simulink model "NDT_Localization"  (R2022a)
settings: Solver=FixedStepAuto  StartTime=0.0  StopTime=10.0  RelTol=1e-3
model workspace (MAT data in the model file):
  SL_ROS_VariableLengthArrays_MaxSizes : object (value not decoded)
undefined symbols (not defined in the file or in its folder): null
libraries: ros2lib x9, robotlib x8, simulink x1
(part 2 of 12)

== system NDT_Localization/observation_callback/check_localizer/If Action Subsystem/register_measurement_impl/If Action Subsystem ==
  message_time : Inport
  ob_msg : Inport  Port=2
  ob_msg_data : Inport  Port=3
  initial_guess : Inport  Port=4
  m_map.frame_id() : Inport  Port=5
  m_map : Inport  Port=6
  localizer_ptr : Inport  Port=7
  Action Port : ActionPort  ActionPortLabel=if(u1 >= u2)
  If : If  IfExpression=u1 == 1  ShowElse=off
  If Action Subsystem : Subsystem  TreatAsAtomicUnit=on
  Merge : Merge
  validate_guess : Subsystem
  summary : Outport
  pose_out : Outport  Port=2
  Out1 : Outport  Port=3
  wires:
  message_time/1 -> If Action Subsystem/1(message_time), validate_guess/1(message_time)
  initial_guess/1 -> If Action Subsystem/2(initial_guess), validate_guess/2(initial_guess)
  validate_guess/1(Out1) -> Merge/1, If/1
  If/1 -> If Action Subsystem/Action
  ob_msg/1 -> If Action Subsystem/3(ob_msg)
  m_map/1 -> If Action Subsystem/5(m_map)
  m_map.frame_id()/1 -> If Action Subsystem/6(m_map.frame_id())
  ob_msg_data/1 -> If Action Subsystem/4(ob_msg_data)
  If Action Subsystem/1(summary) -> summary/1
  If Action Subsystem/2(pose_out) -> pose_out/1
  If Action Subsystem/3(Out2) -> Merge/2
  Merge/1 -> Out1/1
  localizer_ptr/1 -> If Action Subsystem/7(localizer_ptr)

== system NDT_Localization/observation_callback/check_localizer/If Action Subsystem/register_measurement_impl/If Action Subsystem1 ==
  Action Port : ActionPort  ActionPortLabel=else
  Constant : Constant  Value=0
  Out1 : Outport
  wires:
  Constant/1 -> Out1/1

== system NDT_Localization/observation_callback/check_localizer/If Action Subsystem/register_measurement_impl/validate_msg ==
  observation_time : Inport
  m_map : Inport  Port=2
  Add : Sum
  Bus Selector : BusSelector  OutputSignals=stamp.sec,stamp.nanosec
  Constant : Constant  Value=9
  If : If  NumInputs=2  IfExpression=u1 >= u2
  Math Function : Math  Operator=10^u
  Product : Product
  Out1 : Outport
  Out2 : Outport  Port=2
  wires:
  Add/1 -> If/2  "observation_time"
  Math Function/1 -> Product/2
  Constant/1 -> Math Function/1
  Product/1 -> Add/1
  Bus Selector/1 -> Product/1  "<sec>"
  observation_time/1 -> If/1
  Bus Selector/2 -> Add/2  "<nanosec>"
  m_map/1 -> Bus Selector/1
  If/2 -> Out2/1
  If/1 -> Out1/1

== system NDT_Localization/observation_callback/check_localizer/If Action Subsystem/validate_output/If Action Subsystem ==
  pose_out : Inport
  initial_guess : Inport  Port=2
  Action Port : ActionPort  ActionPortLabel=if(u1 ~= 0)
  Out1 : Outport
  wires:
  pose_out/1 -> Out1/1

== system NDT_Localization/observation_callback/check_localizer/If Action Subsystem/validate_output/If Action Subsystem1 ==
  pose_out : Inport
  initial_guess : Inport  Port=2
  Action Port : ActionPort  ActionPortLabel=if(u1 ~= 0)
  Out1 : Outport
  wires:
  pose_out/1 -> Out1/1

== system NDT_Localization/observation_callback/check_localizer/If Action Subsystem/validate_output/Switch Case Action Subsystem ==
  Action Port : ActionPort  ActionPortLabel=case [ 2 ]:
  ret_in : Constant  Value=false
  ret : Outport
  wires:
  ret_in/1 -> ret/1

== system NDT_Localization/observation_callback/check_localizer/If Action Subsystem/validate_output/Switch Case Action Subsystem1 ==
  summary : Inport
  pose_out : Inport  Port=2
  initial_guess : Inport  Port=3
  Action Port : ActionPort  ActionPortLabel=case [ 1 ]:
  Terminator : Terminator
  Terminator1 : Terminator
  Terminator2 : Terminator
  ret_in : Constant  Value=true
  ret : Outport
  wires:
  summary/1 -> Terminator/1
  pose_out/1 -> Terminator1/1
  initial_guess/1 -> Terminator2/1
  ret_in/1 -> ret/1

== system NDT_Localization/observation_callback/check_localizer/If Action Subsystem/validate_output/Switch Case Action Subsystem2 ==
  Action Port : ActionPort  ActionPortLabel=default:
  ret_in : Constant  Value=true
  ret : Outport
  wires:
  ret_in/1 -> ret/1

== system NDT_Localization/map_callback/check_localizer/set_map/set_map_impl/insert/insert_ ==
  msg : Inport
  If : If  NumInputs=2  IfExpression=u1 ~= 0 & u2 ~= 0
  If Action Subsystem : Subsystem  TreatAsAtomicUnit=on
  If Action Subsystem1 : Subsystem  TreatAsAtomicUnit=on
  Merge : Merge
  validate_pcl_map : Subsystem
  insert_res : Outport
  Out2 : Outport  Port=2
  wires:
  msg/1 -> validate_pcl_map/1(msg), If Action Subsystem/1(msg)
  validate_pcl_map/1(Out1) -> If/1
  If/1 -> If Action Subsystem/Action
  If Action Subsystem/1(insert_res) -> insert_res/1
  validate_pcl_map/2(offset) -> If Action Subsystem/2(offset)
  If/2 -> If Action Subsystem1/Action
  If Action Subsystem1/1(Out1) -> Merge/2
  If Action Subsystem/2(Out2) -> Merge/1
  Merge/1 -> Out2/1
  validate_pcl_map/3(ret) -> If/2

== system NDT_Localization/observation_callback/check_localizer/If Action Subsystem/If Action Subsystem/handle_registration_summary/If Action Subsystem ==
  summary : Inport
  Action Port : ActionPort  ActionPortLabel=if(u1 ~= 0)
  Publish : ros2lib/Publish  topicSource=Specify your own  topic=/increment_pub  messageType=sensor_msgs/PointCloud2  QOSHistory=Keep last  QOSDepth=1  QOSReliability=Reliable  QOSDurability=Volatile
      settings: SourceProductBaseCode=RR
  wires:
  summary/1 -> Publish/1

== system NDT_Localization/observation_callback/check_localizer/If Action Subsystem/guess/extrapolate/If Action Subsystem1 ==
  ret : Inport
  Action Port : ActionPort  ActionPortLabel=if(u1 ~= 0)
  Signal Conversion : SignalConversion  OverrideOpt=off
  Out2 : Outport
  wires:
  ret/1 -> Signal Conversion/1
  Signal Conversion/1 -> Out2/1

== system NDT_Localization/observation_callback/check_localizer/If Action Subsystem/guess/extrapolate/lookupTransform ==
  map_frame : Inport
  observation_frame : Inport  Port=2
  If : If  IfExpression=u1 ~= 0
  String Compare : StringCompare
  Switch : Switch  Criteria=u2 > Threshold  SaturateOnIntegerOverflow=off  InputSameDT=off
  TimePointZero : Constant  Value=0
  if_false : Subsystem  TreatAsAtomicUnit=on
  if_true : Subsystem  TreatAsAtomicUnit=on
  ret : Outport
  wires:
  Switch/1 -> ret/1
  map_frame/1 -> String Compare/1, if_false/1(target_frame), if_true/1(target_frame)
  if_true/1(identity) -> Switch/1
  TimePointZero/1 -> if_false/3(time), if_true/3(time)
  If/1 -> if_true/Action
  String Compare/1 -> Switch/2, If/1
  if_false/1(output_transform) -> Switch/3
  If/2 -> if_false/Action
  observation_frame/1 -> if_false/2(source_frame), if_true/2(source_frame), String Compare/2

== system NDT_Localization/observation_callback/check_localizer/If Action Subsystem/guess/lookupTransform/if_false ==
  target_frame : Inport
  source_frame : Inport  Port=2
  time : Inport  Port=3
  Action Port : ActionPort  ActionPortLabel=else
  Bus Creator : BusCreator  Inputs=3
  Bus Creator1 : BusCreator  Inputs=3
  Bus Creator2 : BusCreator  Inputs=2
  Bus Creator3 : BusCreator  Inputs=3
  Bus Creator4 : BusCreator  Inputs=4
  Bus Selector : BusSelector  OutputSignals=time,result_vec.x,result_vec.y,result_vec.z,result_quat.x,result_quat.y,result_quat.z,result_quat.w
  Constant : Constant
  Subsystem : Subsystem
  lookupFrameNumber : Subsystem
  lookupFrameNumber1 : Subsystem
  walkToTopParent : Subsystem  Commented=on
  output_transform : Outport
  wires:
  target_frame/1 -> lookupFrameNumber/1(target_frame), Bus Creator1/3  "frame_id"
  lookupFrameNumber/1(target_id) -> walkToTopParent/3(target_id)
  lookupFrameNumber1/1(source_id) -> walkToTopParent/4(source_id)
  time/1 -> walkToTopParent/2(time)
  Subsystem/1(accum) -> Bus Selector/1, walkToTopParent/1(accum)
  Constant/1 -> Bus Creator1/1  "sec"
  source_frame/1 -> Bus Creator/2, lookupFrameNumber1/1(source_frame)  "child_frame_id"
  Bus Selector/6 -> Bus Creator4/2  "<y>"
  Bus Creator3/1 -> Bus Creator2/1  "translation"
  Bus Selector/8 -> Bus Creator4/4  "<w>"
  Bus Creator4/1 -> Bus Creator2/2  "rotation"
  Bus Creator2/1 -> Bus Creator/3  "transform"
  Bus Creator1/1 -> Bus Creator/1  "header"
  Bus Selector/3 -> Bus Creator3/2  "<y>"
  Bus Selector/5 -> Bus Creator4/1  "<x>"
  Bus Selector/7 -> Bus Creator4/3  "<z>"
  Bus Creator/1 -> output_transform/1
  Bus Selector/1 -> Bus Creator1/2  "<time>"
  Bus Selector/2 -> Bus Creator3/1  "<x>"
  Bus Selector/4 -> Bus Creator3/3  "<z>"

== system NDT_Localization/observation_callback/check_localizer/If Action Subsystem/guess/lookupTransform/if_true ==
  target_frame : Inport
  source_frame : Inport  Port=2
  time : Inport  Port=3
  Action Port : ActionPort  ActionPortLabel=if(u1 ~= 0)
  Bus Creator : BusCreator  Inputs=3
  Bus Creator1 : BusCreator  Inputs=3
  Bus Creator2 : BusCreator  Inputs=2
  Bus Creator3 : BusCreator  Inputs=3
  Bus Creator4 : BusCreator  Inputs=4
  Constant : Constant  Value=false  OutDataTypeStr=boolean
  Current Time : robotlib/Current Time  Commented=on  OutputFormat=bus  SampleTime=-1  ModelName=NDT_Localization
      settings: SourceProductBaseCode=RR
  If : If  NumInputs=2  IfExpression=u1 == u2
  If Action Subsystem : Subsystem  TreatAsAtomicUnit=on
  If Action Subsystem1 : Subsystem  TreatAsAtomicUnit=on
  Merge : Merge
  Switch : Switch  Criteria=u2 > Threshold  SaturateOnIntegerOverflow=off  InputSameDT=off
  getFrame : Subsystem
  getLatestTimestamp : Subsystem
  lookupFrameNumber : Subsystem
  sec : Constant  Value=0  OutDataTypeStr=uint32
  w : Constant  OutDataTypeStr=single
  x : Constant  Value=0  OutDataTypeStr=single
  x1 : Constant  Value=0  OutDataTypeStr=single
  y : Constant  Value=0  OutDataTypeStr=single
  y1 : Constant  Value=0  OutDataTypeStr=single
  z : Constant  Value=0  OutDataTypeStr=single
  z1 : Constant  Value=0  OutDataTypeStr=single
  identity : Outport
  wires:
  Bus Creator1/1 -> Bus Creator/1  "header"
  sec/1 -> Bus Creator1/1  "sec"
  Bus Creator/1 -> identity/1
  source_frame/1 -> Bus Creator/2  "child_frame_id"
  Bus Creator2/1 -> Bus Creator/3  "transform"
  Bus Creator3/1 -> Bus Creator2/1  "translation"
  Bus Creator4/1 -> Bus Creator2/2  "rotation"
  Switch/1 -> Bus Creator1/2  "stamp"
  target_frame/1 -> Bus Creator1/3, lookupFrameNumber/1(target_frame)  "frame_id"
  x/1 -> Bus Creator3/1  "x"
  y/1 -> Bus Creator3/2  "y"
  z/1 -> Bus Creator3/3  "z"
  z1/1 -> Bus Creator4/3  "z"
  y1/1 -> Bus Creator4/2  "y"
  x1/1 -> Bus Creator4/1  "x"
  w/1 -> Bus Creator4/4  "w"
  time/1 -> Switch/3, If/1
  Current Time/1 -> If/2
  If/2 -> If Action Subsystem/Action
  If/1 -> If Action Subsystem1/Action
  If Action Subsystem1/1(out1) -> Merge/1
  If Action Subsystem/1(Out1) -> Merge/2
  Merge/1 -> Switch/2
  Constant/1 -> If Action Subsystem/1(In1)
  lookupFrameNumber/1(target_id) -> getFrame/1(target_id)
  getFrame/1(cache) -> If Action Subsystem1/1(cache), getLatestTimestamp/1(cache)
  getLatestTimestamp/1(LatestTimestamp) -> Switch/1

== system NDT_Localization/observation_callback/check_localizer/If Action Subsystem/register_measurement_impl/If Action Subsystem/If Action Subsystem ==
  message_time : Inport
  initial_guess : Inport  Port=2
  ob_msg : Inport  Port=3
  ob_msg_data : Inport  Port=4
  m_map : Inport  Port=5
  m_map.frame_id() : Inport  Port=6
  localizer_ptr : Inport  Port=7
  Action Port : ActionPort  ActionPortLabel=if(u1 == 1)
  Bus Creator : BusCreator  Inputs=3
  Bus Selector : BusSelector  OutputSignals=OptimizerT.optimizer_options,localizer_config.map_config.voxel_size.x,localizer_config.map_config.voxel_size.y,localizer_config.map_config.voxel_size.z,outlier_ratio
  Bus Selector3 : BusSelector  OutputSignals=transform
  Terminator : Terminator
  Terminator1 : Terminator
  insert : Subsystem
  solve : Subsystem
  transform_to_pose : Subsystem
  transform_to_pose1 : Subsystem
  summary : Outport
  pose_out : Outport  Port=2
  Out2 : Outport  Port=3
  wires:
  initial_guess/1 -> Bus Selector3/1
  Bus Selector3/1 -> transform_to_pose/1(transform_initial_transform)  "<transform>"
  ob_msg/1 -> Terminator/1, insert/2(ob_msg)
  message_time/1 -> insert/1(message_time)
  transform_to_pose/1(eig_pose_initial) -> solve/1(eig_pose_initial)
  insert/1(scan) -> Bus Creator/1  "scan"
  m_map/1 -> Bus Creator/2  "map"
  Bus Selector/5 -> solve/6(outlier_ratio)  "<outlier_ratio>"
  solve/1(summary) -> summary/1
  insert/2(Out2) -> Out2/1
  m_map.frame_id()/1 -> Terminator1/1
  Bus Creator/1 -> solve/2(problem)  "problem"
  ob_msg_data/1 -> insert/3(ob_msg_data)
  solve/2(eig_pose_out) -> transform_to_pose1/1(eig_pose_out)
  transform_to_pose1/1(pose_out.pose.pose) -> pose_out/1
  Bus Selector/2 -> solve/3(voxel_size_x)  "<x>"
  Bus Selector/3 -> solve/4(voxel_size_y)  "<y>"
  Bus Selector/4 -> solve/5(voxel_size_z)  "<z>"
  localizer_ptr/1 -> solve/7(localizer_ptr), Bus Selector/1
  Bus Selector/1 -> Bus Creator/3  "<optimizer_options>"

== system NDT_Localization/observation_callback/check_localizer/If Action Subsystem/register_measurement_impl/If Action Subsystem/validate_guess ==
  message_time : Inport
  initial_guess : Inport  Port=2
  Add : Sum  Inputs=++-  AccumDataTypeStr=uint64
  Bus Selector3 : BusSelector  OutputSignals=header.stamp.sec,header.stamp.nanosec
  Constant : Constant  Value=9
  If : If  NumInputs=2  IfExpression=u1 > u2
  If Action Subsystem : Subsystem  TreatAsAtomicUnit=on
  If Action Subsystem1 : Subsystem  TreatAsAtomicUnit=on
  Math Function : Math  Operator=10^u
  Merge : Merge
  Product : Product
  stamp_tol : Constant  Value=5000  OutDataTypeStr=uint64
  Out1 : Outport
  wires:
  initial_guess/1 -> Bus Selector3/1
  Bus Selector3/1 -> Product/1  "<sec>"
  Bus Selector3/2 -> Add/2  "<nanosec>"
  Product/1 -> Add/1
  Math Function/1 -> Product/2
  Constant/1 -> Math Function/1
  message_time/1 -> Add/3  "message_time"
  Add/1 -> If/1  "guess_scan_diff"
  stamp_tol/1 -> If/2
  If/1 -> If Action Subsystem/Action
  If/2 -> If Action Subsystem1/Action
  If Action Subsystem/1(Out1) -> Merge/1
  If Action Subsystem1/1(Out1) -> Merge/2
  Merge/1 -> Out1/1

== system NDT_Localization/map_callback/check_localizer/set_map/set_map_impl/insert/insert_/If Action Subsystem ==
  msg : Inport
  offset : Inport  Port=2
  Action Port : ActionPort  ActionPortLabel=if(u1 ~= 0)
  While Iterator Subsystem : Subsystem  TreatAsAtomicUnit=on
  insert_res : Outport
  Out2 : Outport  Port=2
  wires:
  msg/1 -> While Iterator Subsystem/1(msg)
  While Iterator Subsystem/1(insert_res) -> insert_res/1
  offset/1 -> While Iterator Subsystem/2(offset)
  While Iterator Subsystem/2(Out2) -> Out2/1

== system NDT_Localization/map_callback/check_localizer/set_map/set_map_impl/insert/insert_/If Action Subsystem1 ==
  Action Port : ActionPort  ActionPortLabel=else
  Constant : Constant  Value=0
  Out1 : Outport
  wires:
  Constant/1 -> Out1/1

== system NDT_Localization/map_callback/check_localizer/set_map/set_map_impl/insert/insert_/validate_pcl_map ==
  msg : Inport
  Add : Sum
  Add1 : Sum
  Add2 : Sum
  Bus Selector : BusSelector  OutputSignals=fields,point_step,height
  Cast : DataTypeConversion  OutDataTypeStr=int8  SaturateOnIntegerOverflow=off  RndMeth=Floor
  Compare To Constant : simulink/Logic and Bit Operations/Compare To Constant  relop=~=  const=1  OutDataTypeStr=boolean
  Constant : Constant  Value=-1
  Constant1 : Constant  Value=-2
  Gain : Gain  Gain=2
  If : If  IfExpression=u1 ~= 0
  If Action Subsystem : Subsystem  TreatAsAtomicUnit=on
  Logical Operator : Logic  Operator=OR  Inputs=3  AllPortsSameDT=off  OutDataTypeStr=boolean
  Merge : Merge
  Product : Product
  Relational Operator : RelationalOperator  Operator=~=  OutDataTypeStr=boolean  RndMeth=Simplest  InputSameDT=off
  Relational Operator1 : RelationalOperator  Operator=~=  OutDataTypeStr=boolean  RndMeth=Simplest  InputSameDT=off
  Width : Width  DataType=uint32
  check_fields : Subsystem  TreatAsAtomicUnit=on
  double_field_size : Constant  Value=8  OutDataTypeStr=uint32
  expected_num_fields : Constant  Value=10
  uint_field_size : Constant  Value=4  OutDataTypeStr=uint32
  Out1 : Outport
  offset : Outport  Port=2
  ret : Outport  Port=3
  wires:
  Bus Selector/1 -> check_fields/1(<fields>), Width/1  "<fields>"
  Logical Operator/1 -> Cast/1
  Product/1 -> Add/1
  double_field_size/1 -> Product/2, check_fields/2(double_field_size)
  Add1/1 -> Product/1
  msg/1 -> check_fields/4(msg), Bus Selector/1
  Bus Selector/3 -> Compare To Constant/1  "<height>"
  Compare To Constant/1 -> Logical Operator/3
  Bus Selector/2 -> Relational Operator1/1  "<point_step>"
  Width/1 -> Relational Operator/2
  Relational Operator1/1 -> Logical Operator/2
  expected_num_fields/1 -> Add2/1, Add1/1, Relational Operator/1
  uint_field_size/1 -> Gain/1
  Gain/1 -> Add/2
  Add/1 -> Relational Operator1/2
  Relational Operator/1 -> Logical Operator/1
  Merge/1 -> Out1/1
  Cast/1 -> If/1
  If/2 -> check_fields/Action
  If/1 -> If Action Subsystem/Action
  If Action Subsystem/1(Out1) -> Merge/1
  Constant/1 -> Add1/2
  Constant1/1 -> Add2/2
  Add2/1 -> check_fields/3(double_field_idx)  "double_field_idx"
  check_fields/1(Out1) -> Merge/2
  check_fields/2(offset) -> offset/1
  check_fields/3(ret) -> ret/1

== system NDT_Localization/observation_callback/check_localizer/If Action Subsystem/guess/extrapolate/lookupTransform/if_false ==
  target_frame : Inport
  source_frame : Inport  Port=2
  time : Inport  Port=3
  Action Port : ActionPort  ActionPortLabel=else
  Bus Creator : BusCreator  Inputs=3
  Bus Creator1 : BusCreator  Inputs=3
  Bus Creator2 : BusCreator  Inputs=2
  Bus Creator3 : BusCreator  Inputs=3
  Bus Creator4 : BusCreator  Inputs=4
  Bus Selector : BusSelector  OutputSignals=time,result_vec.x,result_vec.y,result_vec.z,result_quat.x,result_quat.y,result_quat.z,result_quat.w
  Constant : Constant
  Subsystem : Subsystem
  lookupFrameNumber : Subsystem
  lookupFrameNumber1 : Subsystem
  walkToTopParent : Subsystem  Commented=on
  output_transform : Outport
  wires:
  target_frame/1 -> lookupFrameNumber/1(target_frame), Bus Creator1/3  "frame_id"
  lookupFrameNumber/1(target_id) -> walkToTopParent/3(target_id)
  lookupFrameNumber1/1(source_id) -> walkToTopParent/4(source_id)
  time/1 -> walkToTopParent/2(time)
  Subsystem/1(accum) -> Bus Selector/1, walkToTopParent/1(accum)
  Constant/1 -> Bus Creator1/1  "sec"
  source_frame/1 -> Bus Creator/2, lookupFrameNumber1/1(source_frame)  "child_frame_id"
  Bus Selector/6 -> Bus Creator4/2  "<y>"
  Bus Creator3/1 -> Bus Creator2/1  "translation"
  Bus Selector/8 -> Bus Creator4/4  "<w>"
  Bus Creator4/1 -> Bus Creator2/2  "rotation"
  Bus Creator2/1 -> Bus Creator/3  "transform"
  Bus Creator1/1 -> Bus Creator/1  "header"
  Bus Selector/3 -> Bus Creator3/2  "<y>"
  Bus Selector/5 -> Bus Creator4/1  "<x>"
  Bus Selector/7 -> Bus Creator4/3  "<z>"
  Bus Creator/1 -> output_transform/1
  Bus Selector/1 -> Bus Creator1/2  "<time>"
  Bus Selector/2 -> Bus Creator3/1  "<x>"
  Bus Selector/4 -> Bus Creator3/3  "<z>"

== system NDT_Localization/observation_callback/check_localizer/If Action Subsystem/guess/extrapolate/lookupTransform/if_true ==
  target_frame : Inport
  source_frame : Inport  Port=2
  time : Inport  Port=3
  Action Port : ActionPort  ActionPortLabel=if(u1 ~= 0)
  Bus Creator : BusCreator  Inputs=3
  Bus Creator1 : BusCreator  Inputs=3
  Bus Creator2 : BusCreator  Inputs=2
  Bus Creator3 : BusCreator  Inputs=3
  Bus Creator4 : BusCreator  Inputs=4
  Constant : Constant  Value=false  OutDataTypeStr=boolean
  Current Time : robotlib/Current Time  Commented=on  OutputFormat=bus  SampleTime=-1  ModelName=NDT_Localization
      settings: SourceProductBaseCode=RR
  If : If  NumInputs=2  IfExpression=u1 == u2
  If Action Subsystem : Subsystem  TreatAsAtomicUnit=on
  If Action Subsystem1 : Subsystem  TreatAsAtomicUnit=on
  Merge : Merge
  Switch : Switch  Criteria=u2 > Threshold  SaturateOnIntegerOverflow=off  InputSameDT=off
  getFrame : Subsystem
  getLatestTimestamp : Subsystem
  lookupFrameNumber : Subsystem
  sec : Constant  Value=0  OutDataTypeStr=uint32
  w : Constant  OutDataTypeStr=single
  x : Constant  Value=0  OutDataTypeStr=single
  x1 : Constant  Value=0  OutDataTypeStr=single
  y : Constant  Value=0  OutDataTypeStr=single
  y1 : Constant  Value=0  OutDataTypeStr=single
  z : Constant  Value=0  OutDataTypeStr=single
  z1 : Constant  Value=0  OutDataTypeStr=single
  identity : Outport
  wires:
  Bus Creator1/1 -> Bus Creator/1  "header"
  sec/1 -> Bus Creator1/1  "sec"
  Bus Creator/1 -> identity/1
  source_frame/1 -> Bus Creator/2  "child_frame_id"
  Bus Creator2/1 -> Bus Creator/3  "transform"
  Bus Creator3/1 -> Bus Creator2/1  "translation"
  Bus Creator4/1 -> Bus Creator2/2  "rotation"
  Switch/1 -> Bus Creator1/2  "stamp"
  target_frame/1 -> Bus Creator1/3, lookupFrameNumber/1(target_frame)  "frame_id"
  x/1 -> Bus Creator3/1  "x"
  y/1 -> Bus Creator3/2  "y"
  z/1 -> Bus Creator3/3  "z"
  z1/1 -> Bus Creator4/3  "z"
  y1/1 -> Bus Creator4/2  "y"
  x1/1 -> Bus Creator4/1  "x"
  w/1 -> Bus Creator4/4  "w"
  time/1 -> Switch/3, If/1
  Current Time/1 -> If/2
  If/2 -> If Action Subsystem/Action
  If/1 -> If Action Subsystem1/Action
  If Action Subsystem1/1(out1) -> Merge/1
  If Action Subsystem/1(Out1) -> Merge/2
  Merge/1 -> Switch/2
  Constant/1 -> If Action Subsystem/1(In1)
  lookupFrameNumber/1(target_id) -> getFrame/1(target_id)
  getFrame/1(cache) -> If Action Subsystem1/1(cache), getLatestTimestamp/1(cache)
  getLatestTimestamp/1(LatestTimestamp) -> Switch/1

== system NDT_Localization/observation_callback/check_localizer/If Action Subsystem/guess/lookupTransform/if_false/Subsystem ==
  Bus Creator : BusCreator  Inputs=8
  Bus Creator1 : BusCreator  Inputs=5
  Bus Creator{2,4,6,9} (4 alike) : BusCreator  Inputs=4  OutDataTypeStr=Bus: SL_Bus_geometry_msgs_Quaternion
      settings: InheritFromInputs=off
  Bus Creator{3,5,7..8} (4 alike) : BusCreator  Inputs=3  OutDataTypeStr=Bus: SL_Bus_geometry_msgs_Vector3
      settings: InheritFromInputs=off
  Constant : Constant  OutDataTypeStr=uint32
  Constant1 : Constant  OutDataTypeStr=uint32
  Current Time : robotlib/Current Time  Commented=on  OutputFormat=bus  SampleTime=-1  ModelName=robotlib
      settings: SourceProductBaseCode=RR
  Current Time1 : robotlib/Current Time  Commented=on  OutputFormat=bus  SampleTime=-1  ModelName=robotlib
      settings: SourceProductBaseCode=RR
  w{,1..3} (4 alike) : Constant  OutDataTypeStr=single
  x{,1..7} (8 alike) : Constant  Value=0  OutDataTypeStr=single
  y{,1..7} (8 alike) : Constant  Value=0  OutDataTypeStr=single
  z{,1..7} (8 alike) : Constant  Value=0  OutDataTypeStr=single
  accum : Outport
  wires:
  Bus Creator3/1 -> Bus Creator/4  "source_to_top_vec"
  z4/1 -> Bus Creator6/3  "z"
  z7/1 -> Bus Creator9/3  "z"
  y7/1 -> Bus Creator9/2  "y"
  z1/1 -> Bus Creator4/3  "z"
  y6/1 -> Bus Creator8/2  "y"
  z3/1 -> Bus Creator5/3  "z"
  y1/1 -> Bus Creator4/2  "y"
  w3/1 -> Bus Creator9/4  "w"
  Constant1/1 -> Bus Creator1/5  "child_frame_id_"
  z6/1 -> Bus Creator8/3  "z"
  w/1 -> Bus Creator4/4  "w"
  y/1 -> Bus Creator3/2  "y"
  Bus Creator5/1 -> Bus Creator/6  "terget_to_top_vec"
  y3/1 -> Bus Creator5/2  "y"
  x6/1 -> Bus Creator8/1  "x"
  y4/1 -> Bus Creator6/2  "y"
  Bus Creator6/1 -> Bus Creator/7  "result_quat"
  Bus Creator1/1 -> Bus Creator/1  "st"
  Current Time/1 -> Bus Creator/2  "time"
  x7/1 -> Bus Creator9/1  "x"
  Bus Creator8/1 -> Bus Creator1/2  "translation_"
  Constant/1 -> Bus Creator1/4  "frame_id_"
  y2/1 -> Bus Creator2/2  "y"
  w2/1 -> Bus Creator6/4  "w"
  z2/1 -> Bus Creator2/3  "z"
  Bus Creator4/1 -> Bus Creator/3  "source_to_top_quat"
  x1/1 -> Bus Creator4/1  "x"
  x4/1 -> Bus Creator6/1  "x"
  z/1 -> Bus Creator3/3  "z"
  y5/1 -> Bus Creator7/2  "y"
  x2/1 -> Bus Creator2/1  "x"
  x5/1 -> Bus Creator7/1  "x"
  z5/1 -> Bus Creator7/3  "z"
  Bus Creator7/1 -> Bus Creator/8  "result_vec"
  w1/1 -> Bus Creator2/4  "w"
  x/1 -> Bus Creator3/1  "x"
  Bus Creator2/1 -> Bus Creator/5  "target_to_top_quat"
  Bus Creator9/1 -> Bus Creator1/1  "rotation_"
  Bus Creator/1 -> accum/1  "accum"
  x3/1 -> Bus Creator5/1  "x"
  Current Time1/1 -> Bus Creator1/3  "stamp_"

== system NDT_Localization/observation_callback/check_localizer/If Action Subsystem/guess/lookupTransform/if_false/lookupFrameNumber ==
  target_frame : Inport
  Cast : DataTypeConversion  OutDataTypeStr=uint32  SaturateOnIntegerOverflow=off  RndMeth=Floor
  target_id : Outport
  wires:
  target_frame/1 -> Cast/1
  Cast/1 -> target_id/1

== system NDT_Localization/observation_callback/check_localizer/If Action Subsystem/guess/lookupTransform/if_false/lookupFrameNumber1 ==
  source_frame : Inport
  Cast : DataTypeConversion  OutDataTypeStr=uint32  SaturateOnIntegerOverflow=off  RndMeth=Floor
  source_id : Outport
  wires:
  Cast/1 -> source_id/1
  source_frame/1 -> Cast/1

== system NDT_Localization/observation_callback/check_localizer/If Action Subsystem/guess/lookupTransform/if_false/walkToTopParent ==
  accum : Inport
  time : Inport  Port=2
  target_id : Inport  Port=3
  source_id : Inport  Port=4
  Out1 : Outport

== system NDT_Localization/observation_callback/check_localizer/If Action Subsystem/guess/lookupTransform/if_true/If Action Subsystem ==
  In1 : Inport
  Action Port : ActionPort  ActionPortLabel=else
  Out1 : Outport
  wires:
  In1/1 -> Out1/1

== system NDT_Localization/observation_callback/check_localizer/If Action Subsystem/guess/lookupTransform/if_true/If Action Subsystem1 ==
  cache : Inport
  Action Port : ActionPort  ActionPortLabel=if(u1 == u2)
  Constant : Constant  Commented=on  Value=null
  Constant1 : Constant  Value=true  OutDataTypeStr=boolean
  Constant2 : Constant  Value=false  OutDataTypeStr=boolean
  If : If  NumInputs=2  IfExpression=u1 ~= u2
  If Action Subsystem : Subsystem  TreatAsAtomicUnit=on
  If Action Subsystem1 : Subsystem  TreatAsAtomicUnit=on
  Merge : Merge
  out1 : Outport
  wires:
  Constant/1 -> If/2
  If/1 -> If Action Subsystem/Action
  If/2 -> If Action Subsystem1/Action
  Constant1/1 -> If Action Subsystem/1(In1)
  Constant2/1 -> If Action Subsystem1/1(In1)
  If Action Subsystem/1(Out1) -> Merge/1
  If Action Subsystem1/1(Out1) -> Merge/2
  Merge/1 -> out1/1
  cache/1 -> If/1

== system NDT_Localization/observation_callback/check_localizer/If Action Subsystem/guess/lookupTransform/if_true/getFrame ==
  target_id : Inport
  cache : Outport
  wires:
  target_id/1 -> cache/1

== system NDT_Localization/observation_callback/check_localizer/If Action Subsystem/guess/lookupTransform/if_true/getLatestTimestamp ==
  cache : Inport
  LatestTimestamp : Outport
  wires:
  cache/1 -> LatestTimestamp/1

== system NDT_Localization/observation_callback/check_localizer/If Action Subsystem/guess/lookupTransform/if_true/lookupFrameNumber ==
  target_frame : Inport
  Cast : DataTypeConversion  OutDataTypeStr=uint32  SaturateOnIntegerOverflow=off  RndMeth=Floor
  target_id : Outport
  wires:
  target_frame/1 -> Cast/1
  Cast/1 -> target_id/1

== system NDT_Localization/observation_callback/check_localizer/If Action Subsystem/register_measurement_impl/If Action Subsystem/If Action Subsystem/insert ==
  message_time : Inport
  ob_msg : Inport  Port=2
  ob_msg_data : Inport  Port=3
  Bus Selector : BusSelector  OutputSignals=width
  Constant : Constant  Value=-3
  If : If  NumInputs=2  IfExpression=u1 <= u2
  If Action Subsystem : Subsystem  TreatAsAtomicUnit=on
  If Action Subsystem1 : Subsystem  TreatAsAtomicUnit=on
  Math Function : Math  Operator=10^u
  Merge : Merge
  Product : Product
  Terminator : Terminator
  m_points.capacity : Constant  Value=55000
  scan : Outport
  Out2 : Outport  Port=2
  wires:
  ob_msg/1 -> Bus Selector/1
  message_time/1 -> Product/1
  Math Function/1 -> Product/2
  Constant/1 -> Math Function/1
  Product/1 -> Terminator/1  "m_stamp"
  Bus Selector/1 -> If/1  "<width>"
  If/1 -> If Action Subsystem/Action
  m_points.capacity/1 -> If/2, If Action Subsystem/2(In2)
  If/2 -> If Action Subsystem1/Action
  If Action Subsystem/2(Out2) -> Merge/1
  If Action Subsystem1/1(Out1) -> Merge/2
  Merge/1 -> Out2/1
  If Action Subsystem/1(points) -> scan/1
  ob_msg_data/1 -> If Action Subsystem/1(ob_msg_data)

== system NDT_Localization/observation_callback/check_localizer/If Action Subsystem/register_measurement_impl/If Action Subsystem/If Action Subsystem/solve ==
  eig_pose_initial : Inport
  problem : Inport  Port=2
  voxel_size_x : Inport  Port=3
  voxel_size_y : Inport  Port=4
  voxel_size_z : Inport  Port=5
  outlier_ratio : Inport  Port=6
  localizer_ptr : Inport  Port=7
  Add : Sum  Inputs=+
  Bus Selector : BusSelector  OutputSignals=scan,map,optimizer_options
  Bus Selector1 : BusSelector  OutputSignals=vx.centroid,vx.inv_covariance
  Bus Selector2 : BusSelector  OutputSignals=gradient_tolerance,max_iterations
  For Iterator Subsystem : Subsystem  TreatAsAtomicUnit=on
  If : If  NumInputs=2  IfExpression=u1 <= u2
  If Action Subsystem : Subsystem  TreatAsAtomicUnit=on
  If Action Subsystem1 : Subsystem  TreatAsAtomicUnit=on
  Math Function : Math  Operator=square
  Max : MinMax  Function=max
  Merge1 : Merge
  Product{,1..22} (23 alike) : Product  Multiplication=Matrix(*)
  Terminator : Terminator
  angle_params : Subsystem
  gradient_angle : Subsystem
  hessian_angle : Subsystem
  is_valid_probability : Subsystem  Commented=on
  point_gradient : MATLAB Function  TreatAsAtomicUnit=on
  point_hessian : MATLAB Function  TreatAsAtomicUnit=on
  set_hessian : MATLAB Function  TreatAsAtomicUnit=on
  set_jacobian : MATLAB Function  TreatAsAtomicUnit=on
  summary : Outport
  eig_pose_out : Outport  Port=2
  wires:
  problem/1 -> If Action Subsystem1/1(problem), Bus Selector/1
  Bus Selector/1 -> Product9/1, Product20/1, Product22/1, Product21/1, Product19/1, Product18/1, Product17/1, Product16/1, Product15/1, Product14/1, Product13/1, Product12/1, Product11/1, Product10/1, Product8/1, Product7/1, Product6/1, Product5/1, Product4/1, Product3/1, Product2/1, Product1/1, Product/1, For Iterator Subsystem/1(data)  "<scan>"
  voxel_size_y/1 -> For Iterator Subsystem/6(voxel_size_y), If Action Subsystem1/8(voxel_size_y)
  voxel_size_x/1 -> For Iterator Subsystem/5(voxel_size_x), If Action Subsystem1/7(voxel_size_x)
  voxel_size_z/1 -> If Action Subsystem1/9(voxel_size_z), For Iterator Subsystem/7(voxel_size_z)
  Bus Selector/2 -> Bus Selector1/1  "<map>"
  Bus Selector1/1 -> For Iterator Subsystem/2(myu)  "<centroid>"
  Bus Selector1/2 -> For Iterator Subsystem/3(sigma)  "<inv_covariance>"
  set_jacobian/1(jacobian) -> For Iterator Subsystem/8(set_jacobian)
  point_gradient/1(hessian) -> For Iterator Subsystem/9(set_gradient)
  set_hessian/1(hessian) -> For Iterator Subsystem/10(set_hessian)
  point_hessian/1(hessian) -> For Iterator Subsystem/11(point_hessian)
  angle_params/1(params) -> hessian_angle/1(params), gradient_angle/1(params)
  gradient_angle/1(ga_a_out) -> Product/2
  eig_pose_initial/1 -> If Action Subsystem1/5(eig_pose), angle_params/1(pose)
  Product/1 -> point_gradient/1(ga_a)
  Product1/1 -> point_gradient/2(ga_b)
  Product2/1 -> point_gradient/3(ga_c)
  Product3/1 -> point_gradient/4(ga_d)
  Product4/1 -> point_gradient/5(ga_e)
  gradient_angle/2(ga_b_out) -> Product1/2
  gradient_angle/3(ga_c_out) -> Product2/2
  gradient_angle/4(ga_d_out) -> Product3/2
  gradient_angle/5(ga_e_out) -> Product4/2
  Product5/1 -> point_gradient/6(ga_f)
  gradient_angle/6(ga_f_out) -> Product5/2
  Product6/1 -> point_gradient/7(ga_g)
  gradient_angle/7(ga_g_out) -> Product6/2
  Product7/1 -> point_gradient/8(ga_h)
  gradient_angle/8(ga_h_out) -> Product7/2
  Product8/1 -> point_hessian/1(ha_a2)
  hessian_angle/1(ha_a2_out) -> Product8/2
  Product9/1 -> point_hessian/2(ha_a3)
  hessian_angle/2(ha_a3_out) -> Product9/2
  Product10/1 -> point_hessian/3(ha_b2)
  hessian_angle/3(ha_b2_out) -> Product10/2
  Product11/1 -> point_hessian/4(ha_b3)
  hessian_angle/4(ha_b3_out) -> Product11/2
  Product12/1 -> point_hessian/5(ha_c2)
  hessian_angle/5(ha_c2_out) -> Product12/2
  Product13/1 -> point_hessian/6(ha_c3)
  hessian_angle/6(ha_c3_out) -> Product13/2
  Product14/1 -> point_hessian/7(ha_d1)
  hessian_angle/7(ha_d1_out) -> Product14/2
  Product15/1 -> point_hessian/8(ha_d2)
  hessian_angle/8(ha_d2_out) -> Product15/2
  Product16/1 -> point_hessian/9(ha_d3)
  hessian_angle/9(ha_d3_out) -> Product16/2
  Product17/1 -> point_hessian/10(ha_e1)
  hessian_angle/10(ha_e1_out) -> Product17/2
  Product18/1 -> point_hessian/11(ha_e2)
  hessian_angle/11(ha_e2_out) -> Product18/2
  Product19/1 -> point_hessian/12(ha_e3)
  hessian_angle/12(ha_e3_out) -> Product19/2
  Product20/1 -> point_hessian/13(ha_f1)
  hessian_angle/13(ha_f1_out) -> Product20/2
  Product21/1 -> point_hessian/14(ha_f2)
  hessian_angle/14(ha_f2_out) -> Product21/2
  Product22/1 -> point_hessian/15(ha_f3)
  hessian_angle/15(ha_f3_out) -> Product22/2
  For Iterator Subsystem/2(jacobian_out) -> If Action Subsystem1/2(jacobian), Math Function/1, Max/1
  If/1 -> If Action Subsystem/Action
  If/2 -> If Action Subsystem1/Action
  Bus Selector/3 -> Bus Selector2/1  "<optimizer_options>"
  Bus Selector2/1 -> If/2  "<gradient_tolerance>"
  Math Function/1 -> Add/1
  Add/1 -> If Action Subsystem/1(jacobian)
  Max/1 -> If/1
  If Action Subsystem/1(Out1) -> Merge1/1
  If Action Subsystem1/1(summary) -> Merge1/2
  Merge1/1 -> summary/1
  Bus Selector2/2 -> If Action Subsystem1/4(Max_iter)  "<max_iterations>"
  For Iterator Subsystem/3(hessian_out) -> If Action Subsystem1/3(hessian)
  For Iterator Subsystem/1(score_out) -> Terminator/1
  outlier_ratio/1 -> If Action Subsystem1/6(outlier_ratio), For Iterator Subsystem/4(outlier_ratio)
  If Action Subsystem1/2(eig_pose_result) -> eig_pose_out/1
  localizer_ptr/1 -> If Action Subsystem1/10(localizer_ptr)

== system NDT_Localization/observation_callback/check_localizer/If Action Subsystem/register_measurement_impl/If Action Subsystem/If Action Subsystem/transform_to_pose ==
  transform_initial_transform : Inport
  Add{,1..2,5,7} (5 alike) : Sum
  Add3 : Sum  Inputs=+-
  Add4 : Sum  Inputs=+-
  Add6 : Sum  Inputs=+-
  Asin : Trigonometry  Operator=asin
  Atan1 : Trigonometry  Operator=atan2
  Atan2 : Trigonometry  Operator=atan2
  Bus Selector : BusSelector  OutputSignals=translation,quaternion
  Bus Selector1 : BusSelector  OutputSignals=quaternion_w,quaternion_x,quaternion_y,quaternion_z
  Bus Selector2 : BusSelector  OutputSignals=translation_x,translation_y,translation_z
  Constant : Constant  Value=-2
  Constant1 : Constant  Value=2
  Constant2 : Constant
  Constant3 : Constant  Value=57.3
  Constant4 : Constant  Value=-1
  Constant5 : Constant  Value=pi/180
  Display : Display
  Divide : Product  Inputs=**
  Divide1 : Product  Inputs=**
  Divide2 : Product  Inputs=**
  Matrix Concatenate : Concatenate  NumInputs=6  Mode=Multidimensional array
  Product{,1,7..8} (4 alike) : Product  Inputs=3
  Product{2..6,9..12} (9 alike) : Product
  Square{,1..3} (4 alike) : Math  Operator=square  SignedPower=on
  eig_pose_initial : Outport  VectorParamsAs1DForOutWhenUnconnected=off
  wires:
  Bus Selector2/1 -> Matrix Concatenate/1  "<translation_x>"
  Bus Selector2/2 -> Matrix Concatenate/2  "<translation_y>"
  Bus Selector2/3 -> Matrix Concatenate/3  "<translation_z>"
  Add2/1 -> Add3/1
  Add7/1 -> Atan1/2
  Add1/1 -> Product5/2
  Bus Selector1/2 -> Product8/3, Square2/1, Product3/1  "<quaternion_x>"
  Product11/1 -> Divide/1
  Product12/1 -> Divide2/1
  Product1/1 -> Add/2
  Product3/1 -> Add1/1
  Atan2/1 -> Product6/2
  Atan1/1 -> Product11/2
  Divide/1 -> Matrix Concatenate/4
  Product10/1 -> Add6/2
  Product4/1 -> Add1/2
  Bus Selector1/3 -> Product7/2, Square1/1, Product3/2, Product1/3  "<quaternion_y>"
  Constant4/1 -> Product12/2
  Product9/1 -> Add6/1
  Product8/1 -> Add5/2
  Product6/1 -> Product12/1
  Add/1 -> Asin/1
  Product5/1 -> Atan2/1
  Bus Selector1/1 -> Product8/2, Square3/1, Product4/1, Product1/2, Product/2  "<quaternion_w>"
  Bus Selector1/4 -> Product7/3, Square/1, Product4/2, Product/3  "<quaternion_z>"
  Constant1/1 -> Product8/1, Product7/1, Product10/1, Product5/1, Product1/1
  Add4/1 -> Atan2/2
  Constant/1 -> Product9/1, Product/1
  Constant3/1 -> Product2/1, Product6/1, Product11/1
  Product7/1 -> Add5/1
  Constant5/1 -> Divide/2, Divide2/2, Divide1/2
  Divide1/1 -> Matrix Concatenate/5
  Product2/1 -> Divide1/1
  Add3/1 -> Add4/1
  Divide2/1 -> Matrix Concatenate/6
  Add6/1 -> Add7/2
  Product/1 -> Add/1
  Square/1 -> Add4/2
  Asin/1 -> Product2/2
  Add5/1 -> Atan1/1
  Square2/1 -> Product9/2, Add2/2
  Constant2/1 -> Add7/1
  Square3/1 -> Add2/1
  Square1/1 -> Product10/2, Add3/2
  Matrix Concatenate/1 -> Display/1, eig_pose_initial/1
  transform_initial_transform/1 -> Bus Selector/1
  Bus Selector/2 -> Bus Selector1/1  "<quaternion>"
  Bus Selector/1 -> Bus Selector2/1  "<translation>"

== system NDT_Localization/observation_callback/check_localizer/If Action Subsystem/register_measurement_impl/If Action Subsystem/If Action Subsystem/transform_to_pose1 ==
  eig_pose_out : Inport
  Add{,1..2,5,7} (5 alike) : Sum
  Add3 : Sum  Inputs=+-
  Add4 : Sum  Inputs=+-
  Add6 : Sum  Inputs=+-
  Asin : Trigonometry  Operator=asin
  Atan1 : Trigonometry  Operator=atan2
  Atan2 : Trigonometry  Operator=atan2
  Bus Selector : BusSelector  OutputSignals=translation,quaternion
  Bus Selector1 : BusSelector  OutputSignals=quaternion_w,quaternion_x,quaternion_y,quaternion_z
  Bus Selector2 : BusSelector  OutputSignals=translation_x,translation_y,translation_z
  Constant : Constant  Value=-2
  Constant1 : Constant  Value=2
  Constant2 : Constant
  Constant3 : Constant  Value=57.3
  Constant4 : Constant  Value=-1
  Constant5 : Constant  Value=pi/180
  Display : Display
  Divide : Product  Inputs=**
  Divide1 : Product  Inputs=**
  Divide2 : Product  Inputs=**
  Matrix Concatenate : Concatenate  NumInputs=6  Mode=Multidimensional array
  Product{,1,7..8} (4 alike) : Product  Inputs=3
  Product{2..6,9..12} (9 alike) : Product
  Square{,1..3} (4 alike) : Math  Operator=square  SignedPower=on
  pose_out.pose.pose : Outport  VectorParamsAs1DForOutWhenUnconnected=off
  wires:
  Bus Selector2/1 -> Matrix Concatenate/1  "<translation_x>"
  Bus Selector2/2 -> Matrix Concatenate/2  "<translation_y>"
  Bus Selector2/3 -> Matrix Concatenate/3  "<translation_z>"
  Add2/1 -> Add3/1
  Add7/1 -> Atan1/2
  Add1/1 -> Product5/2
  Bus Selector1/2 -> Product8/3, Square2/1, Product3/1  "<quaternion_x>"
  Product11/1 -> Divide/1
  Product12/1 -> Divide2/1
  Product1/1 -> Add/2
  Product3/1 -> Add1/1
  Atan2/1 -> Product6/2
  Atan1/1 -> Product11/2
  Divide/1 -> Matrix Concatenate/4
  Product10/1 -> Add6/2
  Product4/1 -> Add1/2
  Bus Selector1/3 -> Product7/2, Square1/1, Product3/2, Product1/3  "<quaternion_y>"
  Constant4/1 -> Product12/2
  Product9/1 -> Add6/1
  Product8/1 -> Add5/2
  Product6/1 -> Product12/1
  Add/1 -> Asin/1
  Product5/1 -> Atan2/1
  Bus Selector1/1 -> Product8/2, Square3/1, Product4/1, Product1/2, Product/2  "<quaternion_w>"
  Bus Selector1/4 -> Product7/3, Square/1, Product4/2, Product/3  "<quaternion_z>"
  Constant1/1 -> Product8/1, Product7/1, Product10/1, Product5/1, Product1/1
  Add4/1 -> Atan2/2
  Constant/1 -> Product9/1, Product/1
  Constant3/1 -> Product2/1, Product6/1, Product11/1
  Product7/1 -> Add5/1
  Constant5/1 -> Divide/2, Divide2/2, Divide1/2
  Divide1/1 -> Matrix Concatenate/5
  Product2/1 -> Divide1/1
  Add3/1 -> Add4/1
  Divide2/1 -> Matrix Concatenate/6
  Add6/1 -> Add7/2
  Product/1 -> Add/1
  Square/1 -> Add4/2
  Asin/1 -> Product2/2
  Add5/1 -> Atan1/1
  Square2/1 -> Product9/2, Add2/2
  Constant2/1 -> Add7/1
  Square3/1 -> Add2/1
  Square1/1 -> Product10/2, Add3/2
  Matrix Concatenate/1 -> Display/1, pose_out.pose.pose/1
  eig_pose_out/1 -> Bus Selector/1
  Bus Selector/2 -> Bus Selector1/1  "<quaternion>"
  Bus Selector/1 -> Bus Selector2/1  "<translation>"

== system NDT_Localization/observation_callback/check_localizer/If Action Subsystem/register_measurement_impl/If Action Subsystem/validate_guess/If Action Subsystem ==
  Action Port : ActionPort  ActionPortLabel=if(u1 > u2)
  Constant : Constant  Value=0
  Out1 : Outport
  wires:
  Constant/1 -> Out1/1

== system NDT_Localization/observation_callback/check_localizer/If Action Subsystem/register_measurement_impl/If Action Subsystem/validate_guess/If Action Subsystem1 ==
  Action Port : ActionPort  ActionPortLabel=else
  Constant : Constant
  Out1 : Outport
  wires:
  Constant/1 -> Out1/1

== system NDT_Localization/map_callback/check_localizer/set_map/set_map_impl/insert/insert_/If Action Subsystem/While Iterator Subsystem ==
  msg : Inport
  offset : Inport  Port=2
  Add : Sum
  Bus Creator : BusCreator  Inputs=2
  Bus Selector : BusSelector  OutputSignals=row_step,point_step,header.stamp
  Constant : Constant
  Data Type Conversion : DataTypeConversion  OutDataTypeStr=uint8  SaturateOnIntegerOverflow=off  RndMeth=Floor
  Data Type Conversion{1..3,5..6,9} (6 alike) : DataTypeConversion  OutDataTypeStr=double  SaturateOnIntegerOverflow=off  RndMeth=Floor
  Delay : Delay  DelayLength=1
  If : If  IfExpression=u1 ~= 0
  If Action Subsystem : Subsystem  TreatAsAtomicUnit=on
  If Action Subsystem1 : Subsystem  TreatAsAtomicUnit=on
  MATLAB Function : MATLAB Function  TreatAsAtomicUnit=on
  MATLAB Function1 : MATLAB Function  TreatAsAtomicUnit=on
  MATLAB Function2 : MATLAB Function  TreatAsAtomicUnit=on
  Merge : Merge
  Read Point Cloud : ros2lib/Read Point Cloud  MaximumPointCloudSize=[480, 640]  PreserveStructure=off  ShowRGBOutput=off  ShowIntensityOutput=off  ShowErrorCodeOutput=off  VariableSizeOutputs=off
      settings: SourceProductBaseCode=RR
  Relational Operator : RelationalOperator  Operator=~=  OutDataTypeStr=boolean  RndMeth=Simplest  InputSameDT=off
  Relational Operator1 : RelationalOperator  Operator=~=  OutDataTypeStr=boolean  RndMeth=Simplest  InputSameDT=off
  Relational Operator2 : RelationalOperator  Operator===  OutDataTypeStr=boolean  RndMeth=Simplest  InputSameDT=off
  While Iterator : WhileIterator  MaxIters=55000  ShowIterationPort=on  OutputDataType=uint32
  index : Subsystem
  insert_res : Outport
  Out2 : Outport  Port=2
  wires:
  Relational Operator/1 -> While Iterator/2
  msg/1 -> MATLAB Function/1(msg), Bus Selector/1
  Bus Selector/1 -> Relational Operator/1, Relational Operator1/2  "<row_step>"
  Constant/1 -> Relational Operator/2, Add/2
  Relational Operator1/1 -> While Iterator/1
  While Iterator/1 -> Delay/1, MATLAB Function/2(id), Relational Operator2/2
  Add/1 -> Relational Operator1/1
  Delay/1 -> Add/1
  MATLAB Function/1(point) -> MATLAB Function1/1(point), Read Point Cloud/1
  Read Point Cloud/1 -> Bus Creator/1, index/1(pt)  "centroid"
  index/1(idx) -> If Action Subsystem/1(voxel_idx), Relational Operator2/1  "voxel_idx"
  Relational Operator2/1 -> Data Type Conversion/1
  Data Type Conversion/1 -> If/1
  If/1 -> If Action Subsystem/Action
  If Action Subsystem/1(insert_res) -> insert_res/1
  MATLAB Function2/1(inv_covariance) -> Bus Creator/2  "inv_covariance"
  Bus Creator/1 -> If Action Subsystem/2(vx)  "vx"
  offset/1 -> MATLAB Function1/3(offset)
  Bus Selector/2 -> MATLAB Function1/2(point_step)  "<point_step>"
  MATLAB Function1/1(xx) -> Data Type Conversion1/1
  Data Type Conversion1/1 -> MATLAB Function2/1(xx)
  MATLAB Function1/2(xy) -> Data Type Conversion2/1
  MATLAB Function1/3(xz) -> Data Type Conversion3/1
  MATLAB Function1/4(yy) -> Data Type Conversion5/1
  MATLAB Function1/5(yz) -> Data Type Conversion6/1
  MATLAB Function1/6(zz) -> Data Type Conversion9/1
  Data Type Conversion2/1 -> MATLAB Function2/2(xy)
  Data Type Conversion3/1 -> MATLAB Function2/3(xz)
  Data Type Conversion5/1 -> MATLAB Function2/4(yy)
  Data Type Conversion6/1 -> MATLAB Function2/5(yz)
  Data Type Conversion9/1 -> MATLAB Function2/6(zz)
  If/2 -> If Action Subsystem1/Action
  If Action Subsystem/2(Out2) -> Merge/1
  If Action Subsystem1/1(Out1) -> Merge/2
  Merge/1 -> Out2/1
  Bus Selector/3 -> If Action Subsystem/3(<stamp>)  "<stamp>"

== system NDT_Localization/map_callback/check_localizer/set_map/set_map_impl/insert/insert_/validate_pcl_map/If Action Subsystem ==
  Action Port : ActionPort  ActionPortLabel=if(u1 ~= 0)
  Constant : Constant  Value=0
  Out1 : Outport
  wires:
  Constant/1 -> Out1/1

== system NDT_Localization/map_callback/check_localizer/set_map/set_map_impl/insert/insert_/validate_pcl_map/check_fields ==
  <fields> : Inport
  double_field_size : Inport  Port=2
  double_field_idx : Inport  Port=3
  msg : Inport  Port=4
  Action Port : ActionPort  ActionPortLabel=else
  Cast : DataTypeConversion  OutDataTypeStr=int8  SaturateOnIntegerOverflow=off  RndMeth=Floor
  For Iterator Subsystem : Subsystem  TreatAsAtomicUnit=on
  If : If  IfExpression=u1 ~= 0
  If Action Subsystem : Subsystem  TreatAsAtomicUnit=on
  Logical Operator : Logic  Operator=OR  AllPortsSameDT=off  OutDataTypeStr=boolean
  Merge : Merge
  Subsystem : Subsystem
  Width : Width
  check_fields_name : Subsystem  TreatAsAtomicUnit=on
  Out1 : Outport
  offset : Outport  Port=2
  ret : Outport  Port=3
  wires:
  Logical Operator/1 -> Cast/1
  Cast/1 -> If/1
  If/2 -> check_fields_name/Action
  <fields>/1 -> Width/1, For Iterator Subsystem/2(<fields>), Subsystem/1(<fields>), check_fields_name/1(<fields>)
  If/1 -> If Action Subsystem/Action
  If Action Subsystem/1(Out1) -> Merge/1
  check_fields_name/1(Out1) -> Merge/2
  Merge/1 -> Out1/1
  Width/1 -> For Iterator Subsystem/1(In1)
  double_field_size/1 -> Subsystem/2(double_field_size), For Iterator Subsystem/3(double_field_size)
  double_field_idx/1 -> For Iterator Subsystem/4(double_field_idx)
  For Iterator Subsystem/1(Out1) -> Logical Operator/1
  Subsystem/1(Out1) -> Logical Operator/2
  msg/1 -> check_fields_name/2(msg)
  check_fields_name/2(offset) -> offset/1
  check_fields_name/3(ret) -> ret/1

== system NDT_Localization/observation_callback/check_localizer/If Action Subsystem/guess/extrapolate/lookupTransform/if_false/Subsystem ==
  Bus Creator : BusCreator  Inputs=8
  Bus Creator1 : BusCreator  Inputs=5
  Bus Creator{2,4,6,9} (4 alike) : BusCreator  Inputs=4  OutDataTypeStr=Bus: SL_Bus_geometry_msgs_Quaternion
      settings: InheritFromInputs=off
  Bus Creator{3,5,7..8} (4 alike) : BusCreator  Inputs=3  OutDataTypeStr=Bus: SL_Bus_geometry_msgs_Vector3
      settings: InheritFromInputs=off
  Constant : Constant  OutDataTypeStr=uint32
  Constant1 : Constant  OutDataTypeStr=uint32
  Current Time : robotlib/Current Time  Commented=on  OutputFormat=bus  SampleTime=-1  ModelName=robotlib
      settings: SourceProductBaseCode=RR
  Current Time1 : robotlib/Current Time  Commented=on  OutputFormat=bus  SampleTime=-1  ModelName=robotlib
      settings: SourceProductBaseCode=RR
  w{,1..3} (4 alike) : Constant  OutDataTypeStr=single
  x{,1..7} (8 alike) : Constant  Value=0  OutDataTypeStr=single
  y{,1..7} (8 alike) : Constant  Value=0  OutDataTypeStr=single
  z{,1..7} (8 alike) : Constant  Value=0  OutDataTypeStr=single
  accum : Outport
  wires:
  Bus Creator3/1 -> Bus Creator/4  "source_to_top_vec"
  z4/1 -> Bus Creator6/3  "z"
  z7/1 -> Bus Creator9/3  "z"
  y7/1 -> Bus Creator9/2  "y"
  z1/1 -> Bus Creator4/3  "z"
  y6/1 -> Bus Creator8/2  "y"
  z3/1 -> Bus Creator5/3  "z"
  y1/1 -> Bus Creator4/2  "y"
  w3/1 -> Bus Creator9/4  "w"
  Constant1/1 -> Bus Creator1/5  "child_frame_id_"
  z6/1 -> Bus Creator8/3  "z"
  w/1 -> Bus Creator4/4  "w"
  y/1 -> Bus Creator3/2  "y"
  Bus Creator5/1 -> Bus Creator/6  "terget_to_top_vec"
  y3/1 -> Bus Creator5/2  "y"
  x6/1 -> Bus Creator8/1  "x"
  y4/1 -> Bus Creator6/2  "y"
  Bus Creator6/1 -> Bus Creator/7  "result_quat"
  Bus Creator1/1 -> Bus Creator/1  "st"
  Current Time/1 -> Bus Creator/2  "time"
  x7/1 -> Bus Creator9/1  "x"
  Bus Creator8/1 -> Bus Creator1/2  "translation_"
  Constant/1 -> Bus Creator1/4  "frame_id_"
  y2/1 -> Bus Creator2/2  "y"
  w2/1 -> Bus Creator6/4  "w"
  z2/1 -> Bus Creator2/3  "z"
  Bus Creator4/1 -> Bus Creator/3  "source_to_top_quat"
  x1/1 -> Bus Creator4/1  "x"
  x4/1 -> Bus Creator6/1  "x"
  z/1 -> Bus Creator3/3  "z"
  y5/1 -> Bus Creator7/2  "y"
  x2/1 -> Bus Creator2/1  "x"
  x5/1 -> Bus Creator7/1  "x"
  z5/1 -> Bus Creator7/3  "z"
  Bus Creator7/1 -> Bus Creator/8  "result_vec"
  w1/1 -> Bus Creator2/4  "w"
  x/1 -> Bus Creator3/1  "x"
  Bus Creator2/1 -> Bus Creator/5  "target_to_top_quat"
  Bus Creator9/1 -> Bus Creator1/1  "rotation_"
  Bus Creator/1 -> accum/1  "accum"
  x3/1 -> Bus Creator5/1  "x"
  Current Time1/1 -> Bus Creator1/3  "stamp_"

== system NDT_Localization/observation_callback/check_localizer/If Action Subsystem/guess/extrapolate/lookupTransform/if_false/lookupFrameNumber ==
  target_frame : Inport
  Cast : DataTypeConversion  OutDataTypeStr=uint32  SaturateOnIntegerOverflow=off  RndMeth=Floor
  target_id : Outport
  wires:
  target_frame/1 -> Cast/1
  Cast/1 -> target_id/1

== system NDT_Localization/observation_callback/check_localizer/If Action Subsystem/guess/extrapolate/lookupTransform/if_false/lookupFrameNumber1 ==
  source_frame : Inport
  Cast : DataTypeConversion  OutDataTypeStr=uint32  SaturateOnIntegerOverflow=off  RndMeth=Floor
  source_id : Outport
  wires:
  Cast/1 -> source_id/1
  source_frame/1 -> Cast/1

== system NDT_Localization/observation_callback/check_localizer/If Action Subsystem/guess/extrapolate/lookupTransform/if_false/walkToTopParent ==
  accum : Inport
  time : Inport  Port=2
  target_id : Inport  Port=3
  source_id : Inport  Port=4
  Out1 : Outport
